simulink model "TV_attempt_1"  (R2025a)
settings: Solver=VariableStepAuto  StartTime=0.0  StopTime=10.0  RelTol=1e-3
undefined symbols (not defined in the file): g, L, m, mu
libraries: slpidlib x1
settings Model: Creator=ANITA  LastModifiedBy=ANITA

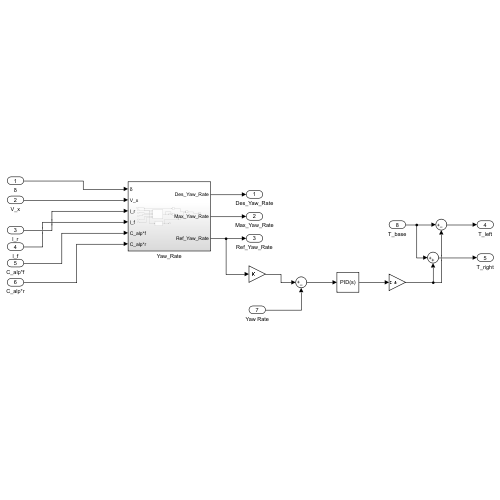
[thumbnail: Simulink's stored preview of the top-level diagram]
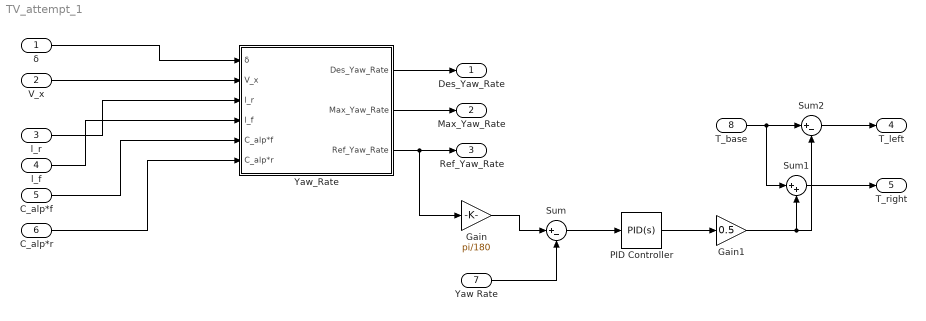
== system TV_attempt_1 ==
  δ : Inport
  V_x : Inport  Port=2
  l_r : Inport  Port=3
  l_f : Inport  Port=4
  C_alp*f : Inport  Port=5
  C_alp*r : Inport  Port=6
  Yaw Rate : Inport  Port=7
  T_base : Inport  Port=8
  Gain : Gain  Gain=pi/180
  Gain1 : Gain  Gain=0.5
  PID Controller : slpidlib/PID Controller  Controller=PID  Form=Parallel  TimeDomain=Continuous-time  UseExternalTs=off  SampleTime=-1  IntegratorMethod=Forward Euler  FilterMethod=Forward Euler  ControllerParametersSource=internal  P=1  I=1  UseKiTs=off  D=0  UseExternalDerivativeSource=off  N=100  UseFilter=on  TunerSelectOption=Transfer Function Based (PID Tuner App)  InitialConditionSource=internal  InitialConditionForIntegrator=0  InitialConditionForFilter=0  DifferentiatorICPrevScaledInput=0  ExternalReset=none  TrackingMode=off  Kt=1  LimitOutput=off  SatLimitsSource=internal  UpperSaturationLimit=inf  LowerSaturationLimit=-inf  LinearizeAsGain=on  AntiWindupMode=none  Kb=1  LimitIntegrator=off  UpperIntegratorSaturationLimit=inf  LowerIntegratorSaturationLimit=-inf  POutMin=[]  POutMax=[]  IOutMin=[]  IOutMax=[]  DOutMin=[]  DOutMax=[]  NOutMin=[]  NOutMax=[]  SumOutMin=[]  SumOutMax=[]  SaturationOutMin=[]  SaturationOutMax=[]  PParamMin=[]  PParamMax=[]  IParamMin=[]  IParamMax=[]  DParamMin=[]  DParamMax=[]  NParamMin=[]  NParamMax=[]  KbParamMin=[]  KbParamMax=[]  KtParamMin=[]  KtParamMax=[]  KbOutMin=[]  KbOutMax=[]  KtOutMin=[]  KtOutMax=[]  IntegratorOutMin=[]  IntegratorOutMax=[]  FilterOutMin=[]  FilterOutMax=[]  SumI1OutMin=[]  SumI1OutMax=[]  SumI2OutMin=[]  SumI2OutMax=[]  SumI3OutMin=[]  SumI3OutMax=[]  SumI4OutMin=[]  SumI4OutMax=[]  SumDOutMin=[]  SumDOutMax=[]  DifferentiatorOutMin=[]  DifferentiatorOutMax=[]  FilterDiffOutCoefMin=[]  FilterDiffOutCoefMax=[]  ReciprocalOutMin=[]  ReciprocalOutMax=[]  SumDenOutMin=[]  SumDenOutMax=[]  SumNumOutMin=[]  SumNumOutMax=[]  DivideOutMin=[]  DivideOutMax=[]  UdiffTsProdOutMin=[]  UdiffTsProdOutMax=[]  NTsProdOutMin=[]  NTsProdOutMax=[]  UintegralTsProdOutMin=[]  UintegralTsProdOutMax=[]  UngainTsProdOutMin=[]  UngainTsProdOutMax=[]  ClampingZeroOutDataTypeStr=Inherit: Inherit via back propagation  ClampingZeroOutMin=[]  ClampingZeroOutMax=[]  FilterDenConstantOutDataTypeStr=Inherit: Inherit via back propagation  FilterDenConstantOutMin=[]  FilterDenConstantOutMax=[]  PCopyOutDataTypeStr=Inherit: Inherit via back propagation  PCopyOutMin=[]  PCopyOutMax=[]  NCopyOutDataTypeStr=Inherit: Inherit via back propagation  NCopyOutMin=[]  NCopyOutMax=[]  IntegratorContinuousStateAttributes=''  IntegratorStateMustResolveToSignalObject=off  IntegratorRTWStateStorageClass=Auto  FilterContinuousStateAttributes=''  FilterStateMustResolveToSignalObject=off  FilterRTWStateStorageClass=Auto  ParallelPVariant=InternalParameters  IdealPVariant=Disabled  IVariant=InternalParameters  DVariant=InternalParameters  IntegratorVariant=Continuous  SatVariant=Disabled  AWVariant=Passthrough  PCopyVariant=Disabled  TRVariant=Disabled  FdbkBlocksVariant=Forward  IdealPFdbkVariant=Disabled  SatFdbkVariant=Disabled  DerivativeFilterVariant=ContFilter  NVariant=InternalParameters  NCopyVariant=Disabled  FilterICVariant=InternalICsFilter  IntegratorICVariant=InternalICs  ExternalResetVariant=Disabled  TRSumVariant=Passthrough  SumFdbkVariant=Disabled  SumVariant=Sum_PID  TsampFilterVariant=InternalTs  TsampNgainVariant=Passthrough  TsampIntegralVariant=Passthrough  ExternalSaturationOutDataTypeStr=Inherit: Same as second input  DerivativeSourceVariant=ErrorSignal  PreIntVariant=InternalPreInt
  Sum : Sum  Inputs=|+-
  Sum1 : Sum  Inputs=|++
  Sum2 : Sum  Inputs=|+-
  Yaw_Rate : Subsystem
  Des_Yaw_Rate : Outport
  Max_Yaw_Rate : Outport  Port=2
  Ref_Yaw_Rate : Outport  Port=3
  T_left : Outport  Port=4
  T_right : Outport  Port=5
  wires:
  δ/1 -> Yaw_Rate/1(δ)
  V_x/1 -> Yaw_Rate/2(V_x)
  l_r/1 -> Yaw_Rate/3(l_r)
  l_f/1 -> Yaw_Rate/4(l_f)
  C_alp*f/1 -> Yaw_Rate/5(C_alp*f)
  C_alp*r/1 -> Yaw_Rate/6(C_alp*r)
  Yaw_Rate/1(Des_Yaw_Rate) -> Des_Yaw_Rate/1
  Yaw_Rate/2(Max_Yaw_Rate) -> Max_Yaw_Rate/1
  Yaw_Rate/3(Ref_Yaw_Rate) -> Gain/1, Ref_Yaw_Rate/1
  Yaw Rate/1 -> Sum/2
  Gain/1 -> Sum/1
  Sum/1 -> PID Controller/1
  PID Controller/1 -> Gain1/1
  Gain1/1 -> Sum2/2, Sum1/2
  T_base/1 -> Sum2/1, Sum1/1
  Sum1/1 -> T_right/1
  Sum2/1 -> T_left/1

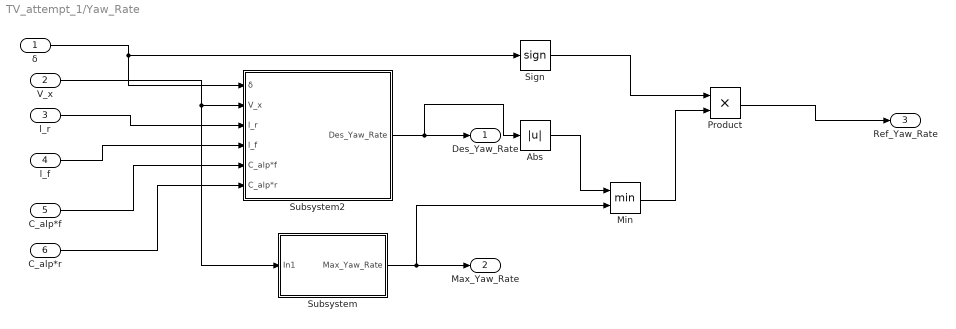
== system TV_attempt_1/Yaw_Rate ==
  δ : Inport
  V_x : Inport  Port=2
  l_r : Inport  Port=3
  l_f : Inport  Port=4
  C_alp*f : Inport  Port=5
  C_alp*r : Inport  Port=6
  Abs : Abs  SaturateOnIntegerOverflow=off
  Min : MinMax  Inputs=2
  Product : Product
  Sign : Signum
  Subsystem : Subsystem
  Subsystem2 : Subsystem
  Des_Yaw_Rate : Outport
  Max_Yaw_Rate : Outport  Port=2
  Ref_Yaw_Rate : Outport  Port=3
  wires:
  δ/1 -> Sign/1, Subsystem2/1(δ)
  l_r/1 -> Subsystem2/3(l_r)
  C_alp*f/1 -> Subsystem2/5(C_alp*f)
  V_x/1 -> Subsystem/1(In1), Subsystem2/2(V_x)
  l_f/1 -> Subsystem2/4(l_f)
  C_alp*r/1 -> Subsystem2/6(C_alp*r)
  Sign/1 -> Product/1
  Subsystem/1(Max_Yaw_Rate) -> Max_Yaw_Rate/1, Min/2
  Product/1 -> Ref_Yaw_Rate/1
  Subsystem2/1(Des_Yaw_Rate) -> Des_Yaw_Rate/1, Abs/1
  Min/1 -> Product/2
  Abs/1 -> Min/1

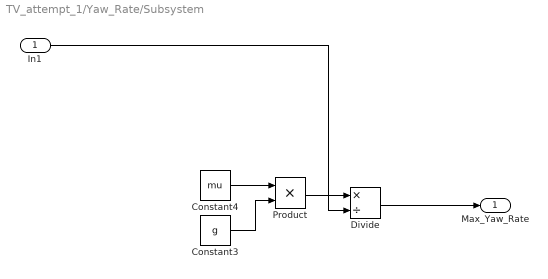
== system TV_attempt_1/Yaw_Rate/Subsystem ==
  In1 : Inport
  Constant3 : Constant  Value=g
  Constant4 : Constant  Value=mu
  Divide : Product  Inputs=*/
  Product : Product
  Max_Yaw_Rate : Outport
  wires:
  Product/1 -> Divide/1
  Divide/1 -> Max_Yaw_Rate/1
  In1/1 -> Divide/2
  Constant3/1 -> Product/2
  Constant4/1 -> Product/1

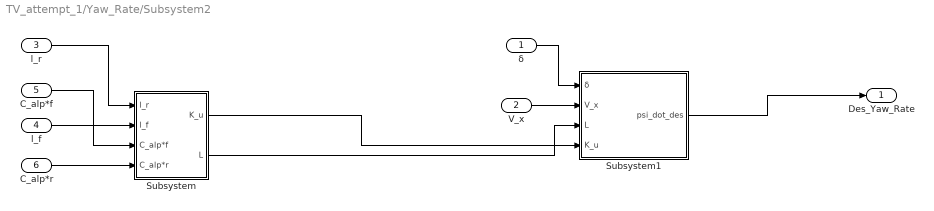
== system TV_attempt_1/Yaw_Rate/Subsystem2 ==
  δ : Inport
  V_x : Inport  Port=2
  l_r : Inport  Port=3
  l_f : Inport  Port=4
  C_alp*f : Inport  Port=5
  C_alp*r : Inport  Port=6
  Subsystem : Subsystem
  Subsystem1 : Subsystem
  Des_Yaw_Rate : Outport
  wires:
  C_alp*f/1 -> Subsystem/3(C_alp*f)
  Subsystem/1(K_u) -> Subsystem1/4(K_u)
  C_alp*r/1 -> Subsystem/4(C_alp*r)
  Subsystem/2(L) -> Subsystem1/3(L)
  l_r/1 -> Subsystem/1(l_r)
  V_x/1 -> Subsystem1/2(V_x)
  l_f/1 -> Subsystem/2(l_f)
  Subsystem1/1(psi_dot_des) -> Des_Yaw_Rate/1
  δ/1 -> Subsystem1/1(δ)

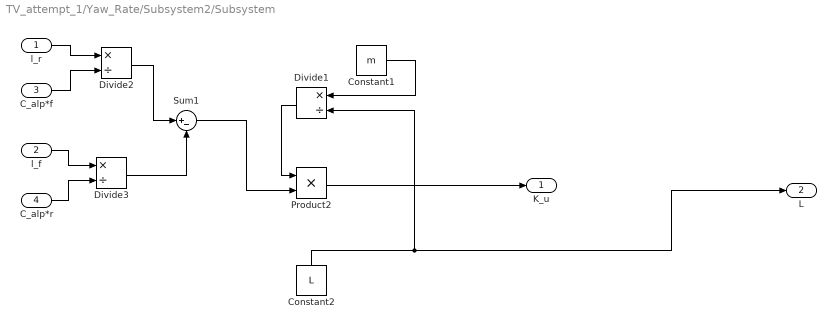
== system TV_attempt_1/Yaw_Rate/Subsystem2/Subsystem ==
  l_r : Inport
  l_f : Inport  Port=2
  C_alp*f : Inport  Port=3
  C_alp*r : Inport  Port=4
  Constant1 : Constant  Value=m
  Constant2 : Constant  Value=L
  Divide1 : Product  Inputs=*/
  Divide2 : Product  Inputs=*/
  Divide3 : Product  Inputs=*/
  Product2 : Product
  Sum1 : Sum  Inputs=|+-
  K_u : Outport
  L : Outport  Port=2
  wires:
  Divide1/1 -> Product2/1
  l_f/1 -> Divide3/1
  Constant2/1 -> L/1, Divide1/2
  Sum1/1 -> Product2/2
  C_alp*r/1 -> Divide3/2
  l_r/1 -> Divide2/1
  Constant1/1 -> Divide1/1
  C_alp*f/1 -> Divide2/2
  Divide2/1 -> Sum1/1
  Divide3/1 -> Sum1/2
  Product2/1 -> K_u/1

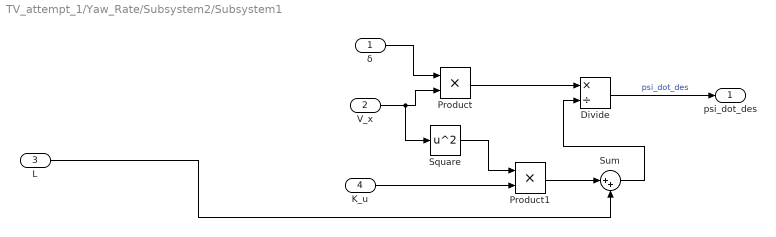
== system TV_attempt_1/Yaw_Rate/Subsystem2/Subsystem1 ==
  δ : Inport
  V_x : Inport  Port=2
  L : Inport  Port=3
  K_u : Inport  Port=4
  Divide : Product  Inputs=*/
  Product : Product
  Product1 : Product
  Square : Math  Operator=square
  Sum : Sum  Inputs=|++
  psi_dot_des : Outport
  wires:
  L/1 -> Sum/2
  Product1/1 -> Sum/1
  V_x/1 -> Square/1, Product/2
  δ/1 -> Product/1
  Product/1 -> Divide/1
  Square/1 -> Product1/1
  Sum/1 -> Divide/2
  K_u/1 -> Product1/2
  Divide/1 -> psi_dot_des/1  "psi_dot_des"
